simulink model "mtdc_droop_control"  (R2016b)
settings: Solver=ode23tb  StartTime=0.0  StopTime=2  RelTol=1e-3  EnableMultiTasking=on
undefined symbols (not defined in the file): sigbuilder_block
libraries: powerlib x22
settings Model: Creator=Amir  LastModifiedBy=Hosein
settings DataIOCC: LimitDataPoints=on  SaveFormat=Array  SignalLoggingSaveFormat=ModelDataLogs
settings OptimizationCC: ExpressionDepthLimit=2147483647  LifeSpan=inf
settings DebuggingCC: UnderspecifiedInitializationDetection=Classic  MergeDetectMultiDrivingBlocksExec=none  SolverPrmCheckMsg=warning  FcnCallInpInsideContextMsg=warning  StateNameClashWarn=warning  StrictBusMsg=Warning  SFUnexpectedBacktrackingDiag=warning  SFNoUnconditionalDefaultTransitionDiag=warning  SFExecutionAtInitializationDiag=none
settings HardwareCC: ProdBitPerPointer=32  ProdBitPerSizeT=32  ProdBitPerPtrDiffT=32  ProdLargestAtomicFloat=None  ProdIntDivRoundTo=Undefined  ProdEndianess=Unspecified  ProdWordSize=32  ProdHWDeviceType=32-bit Generic
settings ModelReferenceCC: PropagateSignalLabelsOutOfModel=off
settings GRTTargetCC: TargetLangStandard=C89/C90 (ANSI)  CombineOutputUpdateFcns=off  GRTInterface=on
settings ConfigComp: CovMetricSettings=dw  CovHtmlReporting=on  CovSaveCumulativeToWorkspaceVar=on  CovSaveSingleToWorkspaceVar=on  CovExternalEMLEnable=off

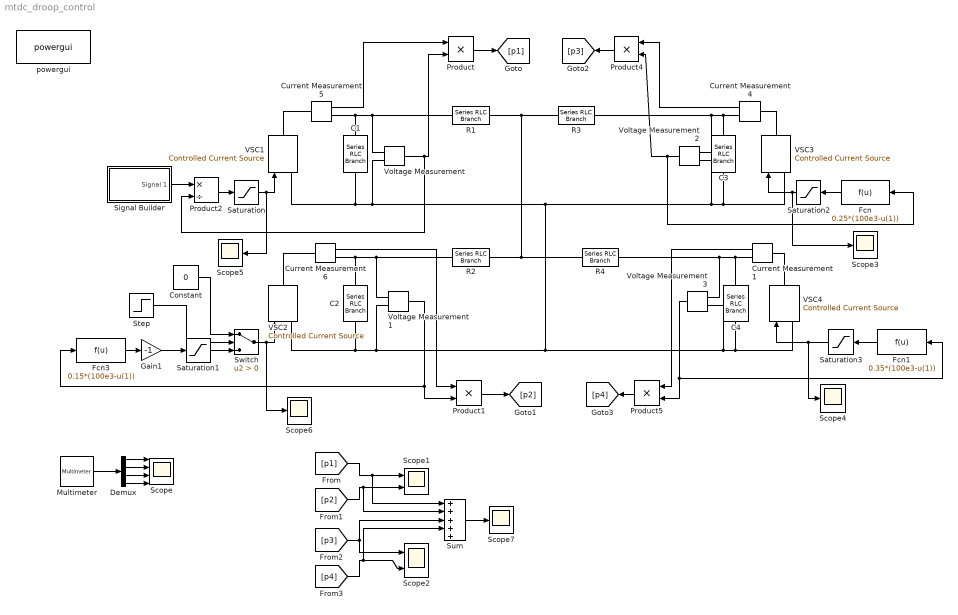
== system mtdc_droop_control ==
  C{1..4} (4 alike) : powerlib/Elements/Series RLC Branch  LConnTagsString=__new0  RConnTagsString=__new0  BranchType=C  Resistance=1  Inductance=1e-3  SetiL0=off  InitialCurrent=0  Capacitance=75e-6  Setx0=on  InitialVoltage=100e3  Measurements=Branch voltage
  Constant : Constant  Value=0
  Current Measurement{1,4..6} (4 alike) : powerlib/Measurements/Current Measurement  PhasorSimulation=off  OutputType=Complex  PSBequivalent=0
  Demux : Demux
  Fcn : Fcn  Expr=0.25*(100e3-u(1))
  Fcn1 : Fcn  Expr=0.35*(100e3-u(1))
  Fcn3 : Fcn  Expr=0.15*(100e3-u(1))
  Gain1 : Gain  Gain=-1
  Multimeter : powerlib/Measurements/Multimeter  PhasorSimulation=off  OutputType=Complex  sel=[1 2 3 4]  L=4  Gain=[1 1 1 1]  yselected={'Ub: C1','Ub: C2','Ub: C3','Ub: C4'};  PSBOutputType=1  PSBequivalent=0  AxesSetting=[0,0.1,-100,100]  Display=0  SavedBlockNames=-11
  Product{,1,4..5} (4 alike) : Product  RndMeth=Zero
  Product2 : Product  Inputs=*/  RndMeth=Zero
  R1 : powerlib/Elements/Series RLC Branch  LConnTagsString=__new0  RConnTagsString=__new0  BranchType=R  Resistance=1.78  Inductance=141.5e-3  SetiL0=off  InitialCurrent=0  Capacitance=1e-6  Setx0=off  InitialVoltage=0  Measurements=None
  R2 : powerlib/Elements/Series RLC Branch  LConnTagsString=__new0  RConnTagsString=__new0  BranchType=R  Resistance=1.78  Inductance=141.5e-3  SetiL0=on  InitialCurrent=-1  Capacitance=1e-6  Setx0=off  InitialVoltage=0  Measurements=None
  R3 : powerlib/Elements/Series RLC Branch  LConnTagsString=__new0  RConnTagsString=__new0  BranchType=R  Resistance=1.78*0.5  Inductance=141.5e-3*0.5  SetiL0=on  InitialCurrent=0.5  Capacitance=1e-6  Setx0=off  InitialVoltage=0  Measurements=None
  R4 : powerlib/Elements/Series RLC Branch  LConnTagsString=__new0  RConnTagsString=__new0  BranchType=R  Resistance=1.78*0.75  Inductance=141.5e-3*0.75  SetiL0=on  InitialCurrent=0.5  Capacitance=1e-6  Setx0=off  InitialVoltage=0  Measurements=None
  Saturation{,1..3} (4 alike) : Saturate  UpperLimit=1000  LowerLimit=-1000
  Scope : Scope  NumInputPorts=4
  Scope1 : Scope  NumInputPorts=2
  Scope2 : Scope  NumInputPorts=2
  Scope{3..7} (5 alike) : Scope
  Signal Builder : Subsystem  Tag=STV Subsys  LoadFcn=sigbuilder_block('load');  StartFcn=sigbuilder_block('start');  StopFcn=sigbuilder_block('stop');  ClipboardFcn=sigbuilder_block('clipboard');  mask(Sigbuilder block){tuvar=[0:10]}
      mask help: Sigbuilder GUI
      mask init:
      | if ~strcmp(get_param(bdroot(gcbh),'SimulationStatus'),'stopped') tuvar = sigbuilder_block('maskInit'); end
      settings: CopyFcn=sigbuilder_block('copy');  DeleteFcn=sigbuilder_block('delete');  ModelCloseFcn=sigbuilder_block('modelClose');  PreSaveFcn=sigbuilder_block('preSave');  PauseFcn=sigbuilder_block('pause')  ContinueFcn=sigbuilder_block('continue')  NameChangeFcn=sigbuilder_block('namechange');  OpenFcn=sigbuilder_block('open',[437.25 199.5 550.5 399.75 ]);  CloseFcn=sigbuilder_block('close');
      mask Display: plot(0,0,100,100,[10,10,40,40,10],[80,20,20,80,80],[40,10],[50,50], [40,27,10],[65,72,56],[40,25,25,10],[28,28,43,43]);
  Step : Step  Time=10  SampleTime=0
  Sum : Sum  Inputs=5
  Switch : Switch  Criteria=u2 > Threshold
  VSC{1..4} (4 alike) : powerlib/Electrical Sources/Controlled Current Source  Initialize=on  Source_Type=AC  Amplitude=0  Phase=0  Frequency=0  Measurements=None
  Voltage Measurement{,1..3} (4 alike) : powerlib/Measurements/Voltage Measurement  PhasorSimulation=off  OutputType=Complex  PSBequivalent=0
  powergui : powerlib/powergui  Priority=1  SimulationMode=Discrete  SolverType=Tustin/Backward Euler (TBE)  SampleTime=1e-4  frequency=60  SPID=off  DisableSnubberDevices=off  DisableRonSwitches=off  DisableVfSwitches=off  SwTol=0  DisplayEquations=off  Interpol=off  ExternalGateDelay=off  methode=off  Ts=0  FunctionMessages=off  echomessages=off  HookPort=off  EnableUseOfTLC=off  x0status=blocks  frequencyindice=0  Pbase=100e6  ErrMax=1e-4  Iterations=50  UnitsV=kV  UnitsW=MW  buscounter=0  RestoreLinks=warning  ResistiveCurrentMeasurement=off  Frange=[0:2:500]  Ylog=off  Xlog=on  ShowGrid=off  save=off  variable=ZData  structure=0  ZoomFFT=on  StartTime=0.0  cycles=1  DisplayStyle=1  fundamental=60  FreqAxis=off  MaxFrequency=1000  frequencyindicesteady=1  RmsSteady=1  display=off
  wires:
  Fcn1/1 -> Saturation3/1
  Fcn/1 -> Saturation2/1
  Fcn3/1 -> Gain1/1
  Multimeter/1 -> Demux/1
  Demux/1 -> Scope/1
  Demux/2 -> Scope/2
  Demux/3 -> Scope/3
  Demux/4 -> Scope/4
  Voltage Measurement/1 -> Product/2, Product2/2
  Current Measurement6/1 -> Product1/1
  Voltage Measurement1/1 -> Product1/2, Fcn3/1
  Product/1 -> [p1]
  Product1/1 -> [p2]
  [p1] -> Scope1/1, Sum/1
  [p2] -> Scope1/2, Sum/2
  Voltage Measurement2/1 -> Product4/2, Fcn/1
  Voltage Measurement3/1 -> Product5/2, Fcn1/1
  Current Measurement4/1 -> Product4/1
  Current Measurement1/1 -> Product5/1
  Product4/1 -> [p3]
  Product5/1 -> [p4]
  [p3] -> Scope2/1, Sum/3
  [p4] -> Sum/4, Scope2/2
  Sum/1 -> Scope7/1
  Current Measurement5/1 -> Product/1
  Signal Builder/1(Signal 1) -> Product2/1
  Product2/1 -> Saturation/1
  Gain1/1 -> Saturation1/1
  Saturation/1 -> VSC1/1, Scope5/1
  Saturation2/1 -> VSC3/1, Scope3/1
  Saturation3/1 -> VSC4/1, Scope4/1
  Switch/1 -> VSC2/1, Scope6/1
  Saturation1/1 -> Switch/3
  Step/1 -> Switch/2
  Constant/1 -> Switch/1
  connections:
  R1/LConn1 -- C1/LConn1 -- Current Measurement5/RConn1 -- Voltage Measurement/LConn1
  VSC4/LConn1 -- C4/RConn1 -- Voltage Measurement3/LConn2 -- VSC1/LConn1 -- C1/RConn1 -- Voltage Measurement/LConn2 -- VSC3/LConn1 -- C3/RConn1 -- Voltage Measurement2/LConn2 -- VSC2/LConn1 -- C2/RConn1 -- Voltage Measurement1/LConn2
  R4/LConn1 -- R1/RConn1 -- R3/LConn1 -- R2/RConn1
  R3/RConn1 -- Voltage Measurement2/LConn1 -- C3/LConn1 -- Current Measurement4/RConn1
  R2/LConn1 -- C2/LConn1 -- Current Measurement6/RConn1 -- Voltage Measurement1/LConn1
  R4/RConn1 -- C4/LConn1 -- Current Measurement1/RConn1 -- Voltage Measurement3/LConn1
  Current Measurement5/LConn1 -- VSC1/RConn1
  Current Measurement6/LConn1 -- VSC2/RConn1
  Current Measurement1/LConn1 -- VSC4/RConn1
  Current Measurement4/LConn1 -- VSC3/RConn1

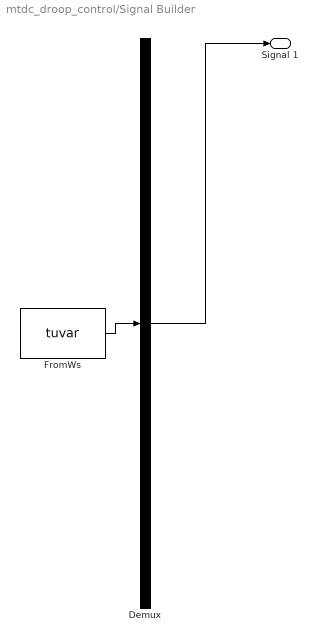
== system mtdc_droop_control/Signal Builder ==
  Demux : Demux  Tag=STV Demux  Outputs=1
  FromWs : FromWorkspace  Tag=STV FromWs  VariableName=tuvar  SampleTime=0
      SigBuilderData=|
      | common.afterFinalStr = 'Extrapolate'
      | common.sampleTime = 0
      | dataSet.timeRange = [0 2]
      | dataSet.name = 'Group 1'
      | sbobj.Groups.Name = 'Group 1'
      | sbobj.Groups.Signals.Name = 'Signal 1'
      | sbobj.Groups.Signals.XData = [0 0.4 0.4 1 1 2]
      | sbobj.Groups.Signals.YData = [50000000 50000000 80500000 80500000 8500000 8500000]
  Signal 1 : Outport  Tag=STV Outport
  wires:
  Demux/1 -> Signal 1/1
  FromWs/1 -> Demux/1
